simulink model "SAT_CONTROL"  (R2018b)
settings: Solver=FixedStepAuto  StartTime=0.0  StopTime=100  FixedStep=0.001  RelTol=1e-3
settings Model: Creator=22672  LastModifiedBy=cx

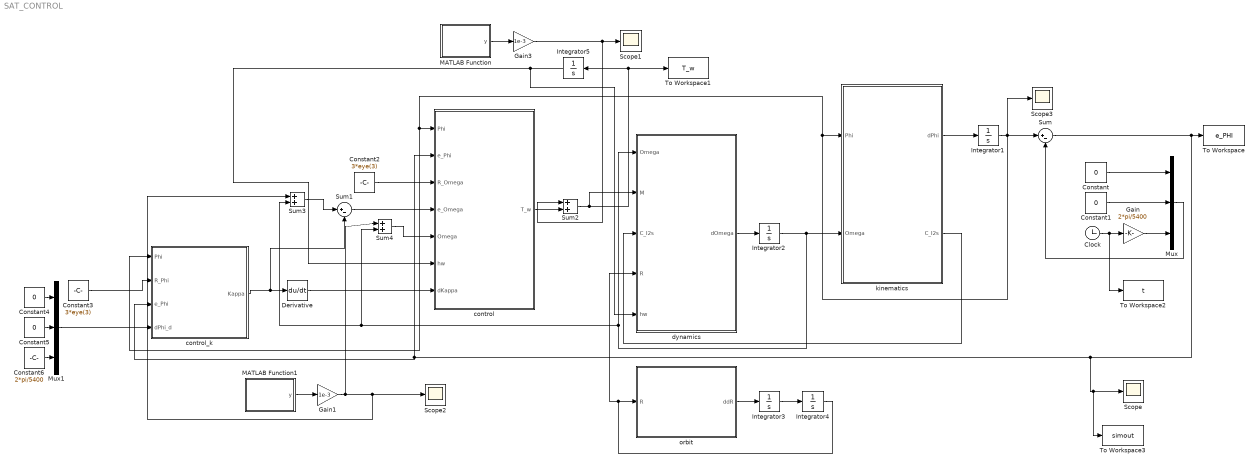
== system SAT_CONTROL ==
  Clock : Clock
  Constant{,1,4..5} (4 alike) : Constant  Value=0
  Constant2 : Constant  Value=3*eye(3)
  Constant3 : Constant  Value=3*eye(3)
  Constant6 : Constant  Value=2*pi/5400
  Derivative : Derivative
  Gain : Gain  Gain=2*pi/5400
  Gain1 : Gain  Gain=1e-3
  Gain3 : Gain  Gain=1e-3
  Integrator1 : Integrator  InitialCondition=[0 0 0]'
  Integrator2 : Integrator  InitialCondition=[0 0 0]'
  Integrator3 : Integrator  InitialCondition=[0 sqrt(3.986e14/6871393) 0]'
  Integrator4 : Integrator  InitialCondition=[6871393 0 0]'
  Integrator5 : Integrator  InitialCondition=[0.0015 0.0015 0.0015]'
  MATLAB Function : MATLAB Function  TreatAsAtomicUnit=on
  MATLAB Function1 : MATLAB Function  TreatAsAtomicUnit=on
  Mux : Mux  Inputs=3
  Mux1 : Mux  Inputs=3
  Scope{,1..3} (4 alike) : Scope
  Sum : Sum  Inputs=|+-
  Sum1 : Sum  Inputs=|+-
  Sum2 : Sum  Inputs=|++
  Sum3 : Sum  Inputs=|++
  Sum4 : Sum  Inputs=|++
  To Workspace : ToWorkspace  VariableName=e_PHI  SampleTime=-1
  To Workspace1 : ToWorkspace  VariableName=T_w  SampleTime=-1
  To Workspace2 : ToWorkspace  VariableName=t  SampleTime=-1
  To Workspace3 : ToWorkspace  VariableName=simout  SaveFormat=Timeseries  SampleTime=-1
  control : MATLAB Function  TreatAsAtomicUnit=on
  control_k : MATLAB Function  TreatAsAtomicUnit=on
  dynamics : MATLAB Function  TreatAsAtomicUnit=on
  kinematics : MATLAB Function  TreatAsAtomicUnit=on
  orbit : MATLAB Function  TreatAsAtomicUnit=on
  wires:
  Constant6/1 -> Mux1/3
  Derivative/1 -> control/7(dKappa)
  Constant1/1 -> Mux/2
  control_k/1(Kappa) -> Sum1/2, Derivative/1
  orbit/1(ddR) -> Integrator3/1
  Integrator5/1 -> dynamics/5(hw), control/6(hw)
  Constant/1 -> Mux/1
  Mux1/1 -> control_k/4(dPhi_d)
  Sum1/1 -> control/4(e_Omega)
  Constant4/1 -> Mux1/1
  Integrator2/1 -> dynamics/1(Omega), Sum4/2, Sum3/2, kinematics/2(Omega)
  kinematics/2(C_I2s) -> dynamics/3(C_I2s)
  Integrator1/1 -> Scope3/1, Sum/1, kinematics/1(Phi), control_k/1(Phi), control/1(Phi)
  Constant5/1 -> Mux1/2
  kinematics/1(dPhi) -> Integrator1/1
  Sum/1 -> To Workspace/1, To Workspace3/1, Scope/1, control/2(e_Phi), control_k/3(e_Phi)
  Clock/1 -> To Workspace2/1, Gain/1
  Constant2/1 -> control/3(R_Omega)
  Integrator3/1 -> Integrator4/1
  Integrator4/1 -> dynamics/4(R), orbit/1(R)
  Mux/1 -> Sum/2
  Gain/1 -> Mux/3
  Constant3/1 -> control_k/2(R_Phi)
  dynamics/1(dOmega) -> Integrator2/1
  MATLAB Function/1(y) -> Gain3/1
  Gain3/1 -> Scope1/1, Sum2/1
  Sum2/1 -> dynamics/2(M), Integrator5/1, To Workspace1/1
  control/1(T_w) -> Sum2/2
  Gain1/1 -> Sum4/1, Sum3/1, Scope2/1
  MATLAB Function1/1(y) -> Gain1/1
  Sum3/1 -> Sum1/1
  Sum4/1 -> control/5(Omega)

== matlab function SAT_CONTROL/orbit ==
  data: ddR output; R input
function ddR  = orbit(R)

mu=3.986e14;
ddR=-mu/norm(R)^2;
end

== matlab function SAT_CONTROL/dynamics ==
  data: Omega input; M input; dOmega output; C_I2s input; R input; hw input
function dOmega   = dynamics(Omega,M,C_I2s,R,hw)
%航天器小角度近似姿态动力学模型 圆轨道假设、小角度假设
%Y = [滚转角速度，偏航角速度，俯仰角速度，滚转角，偏航角，俯仰角]，Cx(滚转) Cz(俯仰) Cy(偏航)
%主轴转动惯量
Ix = 0.533;
Iy = 0.533*2;
Iz = 0.533*3;
J=diag([Ix Iy Iz]);
mu = 3.986e14;%地球引力常数m^3/s^-2
Rs=C_I2s*R;
%动力学模型
Me=3*mu/(norm(Rs)^5)*cross(Rs,J*Rs);
dOmega=J\(-cross(Omega,J*Omega+hw)+M+Me);
end

== matlab function SAT_CONTROL/control ==
  data: Phi input; e_Phi input; R_Omega input; e_Omega input; Omega input; T_w output; hw input; dKappa input
function T_w  = control(Phi,e_Phi,R_Omega,e_Omega,Omega,hw,dKappa)
phi=Phi(1);
theta=Phi(2);
psi=Phi(3);
Ix = 0.533;
Iy = 0.533*2;
Iz = 0.533*3;
J=diag([Ix Iy Iz]);
F=[1 sin(phi)*tan(theta) cos(phi)*tan(theta)
   0 cos(phi) -sin(phi)
   0 sin(phi)/cos(theta) cos(phi)/cos(theta)];
T_w=-F'*e_Phi-R_Omega*e_Omega+cross(Omega,J*Omega+hw)+J*dKappa;
end

== matlab function SAT_CONTROL/control_k ==
  data: Phi input; R_Phi input; e_Phi input; Kappa output; dPhi_d input
function Kappa  = control_k(Phi,R_Phi,e_Phi,dPhi_d)
phi=Phi(1);
theta=Phi(2);
F=[1 sin(phi)*tan(theta) cos(phi)*tan(theta)
   0 cos(phi) -sin(phi)
   0 sin(phi)/cos(theta) cos(phi)/cos(theta)];
Kappa=F\(dPhi_d-R_Phi*e_Phi);
end

== matlab function SAT_CONTROL/MATLAB Function ==
  data: y output
function y = disturb()
y=wgn(1,1,1);

== matlab function SAT_CONTROL/MATLAB Function1 ==
  data: y output
function y = disturb()
y=wgn(1,1,1);

== matlab function SAT_CONTROL/kinematics ==
  data: Phi input; Omega input; dPhi output; C_I2s output
function [dPhi, C_I2s]  = kinematics(Phi,Omega)
phi=Phi(1);
theta=Phi(2);
psi=Phi(3);
F=[1 sin(phi)*tan(theta) cos(phi)*tan(theta)
   0 cos(phi) -sin(phi)
   0 sin(phi)/cos(theta) cos(phi)/cos(theta)];
dPhi=F*Omega;
C_3=[cos(psi) sin(psi) 0
     -sin(psi) cos(psi) 0
     0 0 1];
C_2=[cos(theta) 0 -sin(theta)
     0 1 0
     sin(theta) 0 cos(theta)];
C_1=[1 0 0
     0 cos(phi) sin(phi)
     0 -sin(phi) cos(phi)];
 C_I2s=C_1*C_2*C_3;
end
